simulink model "trasformatore"  (Simulink 10.0)
settings: Solver=ode45  StartTime=0.0  StopTime=10  RelTol=1e-5  EnableMultiTasking=on
values from neighbouring files (symbols this model uses):
  A = Pi*Q    [s_trasformatore.m]
  B = Pi*R    [s_trasformatore.m]
  C = [0 -RL;1 0;0 1]    [s_trasformatore.m]
  D = [0 0 0]'    [s_trasformatore.m]
  x0 = zeros(2,1)    [s_trasformatore.m]
settings Model: Creator=prof. G. Celentano  LastModifiedBy=giuseppericcio  ExtModeTrigMode=oneshot  ExtModeArmWhenConnect=off
settings DataIOCC: SignalLoggingSaveFormat=ModelDataLogs  SignalLoggingName=sigsOut
settings OptimizationCC: BooleanDataType=off  ExpressionDepthLimit=2147483647
settings DebuggingCC: SaveWithParameterizedLinksMsg=none  SignalResolutionControl=TryResolveAllWithWarning  MultiTaskDSMMsg=warning  MultiTaskCondExecSysMsg=none  FcnCallInpInsideContextMsg=warning  StateNameClashWarn=warning
settings HardwareCC: TargetUnknown=on

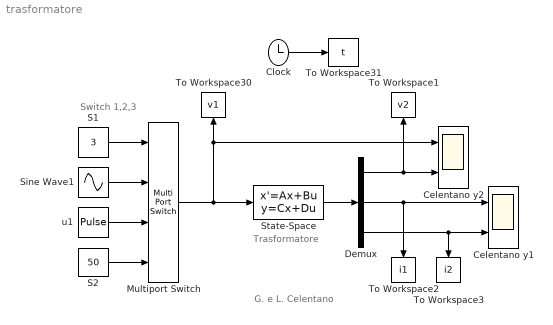
== system trasformatore ==
  note: Switch
      | 1,2,3
  note: G. e L. Celentano
  note: Trasformatore
  Celentano y1 : Scope  NumInputPorts=2
  Celentano y2 : Scope  NumInputPorts=2
  Clock : Clock
  Demux : Demux  Outputs=3
  Multiport Switch : MultiPortSwitch  SaturateOnIntegerOverflow=on  InputSameDT=on
  S1 : Constant  Value=3
  S2 : Constant  Value=50
  Sine Wave1 : Sin  Amplitude=sqrt(2)*220  Frequency=2*pi*50  Phase=pi/4  SampleTime=0
  State-Space : StateSpace  A=A  B=B  C=C  D=D  InitialCondition=x0
  To Workspace1 : ToWorkspace  VariableName=v2  SampleTime=-1
  To Workspace2 : ToWorkspace  VariableName=i1  SampleTime=-1
  To Workspace3 : ToWorkspace  VariableName=i2  SampleTime=-1
  To Workspace30 : ToWorkspace  VariableName=v1  SampleTime=-1
  To Workspace31 : ToWorkspace  VariableName=t  SampleTime=-1
  u1 : DiscretePulseGenerator  PulseType=Time based  Amplitude=100  Period=.02  PulseWidth=50
  wires:
  Multiport Switch/1 -> State-Space/1, Celentano y2/1, To Workspace30/1
  Clock/1 -> To Workspace31/1
  Sine Wave1/1 -> Multiport Switch/2
  S1/1 -> Multiport Switch/1
  State-Space/1 -> Demux/1
  Demux/1 -> Celentano y2/2, To Workspace1/1
  Demux/2 -> Celentano y1/1, To Workspace2/1
  Demux/3 -> Celentano y1/2, To Workspace3/1
  S2/1 -> Multiport Switch/4
  u1/1 -> Multiport Switch/3
